simulink model "PD_vel_controller_for_SOIPTD_parametric"  (R2019b)
settings: Solver=VariableStepAuto  StartTime=0.0  StopTime=10.0  RelTol=1e-3
undefined symbols (not defined in the file or in its folder): D, frequency, K, P, T1, T2, tau
libraries: simulink x1
settings Model: Creator=aaa_b  LastModifiedBy=aaa_b

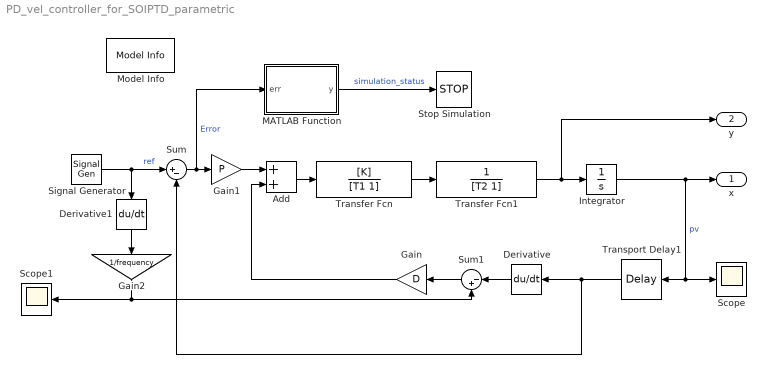
== system PD_vel_controller_for_SOIPTD_parametric ==
  Add : Sum
  Derivative : Derivative
  Derivative1 : Derivative  CoefficientInTFapproximation=0
  Gain : Gain  Gain=D
  Gain1 : Gain  Gain=P
  Gain2 : Gain  Gain=1/frequency
  Integrator : Integrator
  MATLAB Function : MATLAB Function  TreatAsAtomicUnit=on
  Model Info : simulink/Model-Wide Utilities/Model Info  Frame=on  DisplayStringWithTags=Model Info How should we take sensors reading WITHOUT delay  HorizontalTextAlignment=Center  LeftAlignmentValue=0.5
  Scope : Scope
  Scope1 : Scope
  Signal Generator : SignalGenerator  Frequency=frequency  Units=rad/sec
  Stop Simulation : Stop
  Sum : Sum  Inputs=|+-
  Sum1 : Sum  Inputs=|-+
  Transfer Fcn : TransferFcn  Numerator=[K]  Denominator=[T1 1]
  Transfer Fcn1 : TransferFcn  Denominator=[T2 1]
  Transport Delay1 : TransportDelay  DelayTime=tau
  x : Outport  VectorParamsAs1DForOutWhenUnconnected=off
  y : Outport  Port=2  VectorParamsAs1DForOutWhenUnconnected=off
  wires:
  Derivative/1 -> Sum1/1
  Derivative1/1 -> Gain2/1
  Sum1/1 -> Gain/1
  MATLAB Function/1(y) -> Stop Simulation/1  "simulation_status"
  Signal Generator/1 -> Derivative1/1, Sum/1  "ref"
  Transport Delay1/1 -> Sum/2, Derivative/1
  Add/1 -> Transfer Fcn/1
  Sum/1 -> MATLAB Function/1(err), Gain1/1  "Error"
  Transfer Fcn1/1 -> y/1, Integrator/1
  Transfer Fcn/1 -> Transfer Fcn1/1
  Gain/1 -> Add/2
  Integrator/1 -> Scope/1, Transport Delay1/1, x/1  "pv"
  Gain2/1 -> Scope1/1, Sum1/2
  Gain1/1 -> Add/1

== matlab function PD_vel_controller_for_SOIPTD_parametric/MATLAB Function ==
  data: err input; y output
function y = fcn(err)
if (abs(err)>1000)
    y=1;
else
    y=0;
end
